simulink model "model"  (R2021a)
settings: Solver=VariableStepAuto  StartTime=0.0  StopTime=50000  RelTol=1e-3
values from neighbouring files (symbols this model uses):
  C_index = 3    [parameters.m]    (also in parameters.mat)
  C_r = 6.6    [parameters.m]    (also in parameters.mat)
  Capacity_noise = 10    [parameters.m]    (also in parameters.mat)
  cell_count = 12    [parameters.m]    (also in parameters.mat)
  Parameter_noise = 80    [parameters.m]    (also in parameters.mat)
  Q_index = 2    [parameters.m]    (also in parameters.mat)
  Rp = Rp_LUT    [parameters.m]    (also in parameters.mat = [0.0013284973182 0.00132849731829 0.00133071540687 0.0013310)
  Rs = Rs_LUT    [parameters.m]    (also in parameters.mat = [0.0044622496006 0.00446224960062 0.00395928973129 0.0036572)
  soc_LUT = [0, 0.01, 0.0909090909090909,0.181818181818182,0.272727272727273,0.363636363636364,0.454545454545455,0.545454545454545,0.636363636363636,0.727272727272727,0.818181818181818,0.909090909090909,1]    [parameters.m]    (also in parameters.mat = [0 0.01 0.0909090909091 0.181818181818 0.272727272727 0.3636)
  tau = tau_LUT    [parameters.m]    (also in parameters.mat = [950.87194683 950.871946837 952.459545918 952.715608142 956.)
  Ts_macro = 60    [parameters.m]    (also in parameters.mat)
  Ts_micro = 0.02    [parameters.m]    (also in parameters.mat)
  z0 = 0.5    [parameters.m]    (also in parameters.mat)
undefined symbols (not defined in the file or in its folder): awgn, CC_level, CV_level, is_CC, is_CV
libraries: nesl_utility x42, fl_lib x30, ee_lib x12, simulink x11, sharedTrackingLibrary x2, simulink_extras x1
(part 1 of 3)
settings Model: SimulationMode=accelerator  Creator=oscar  LastModifiedBy=oscar

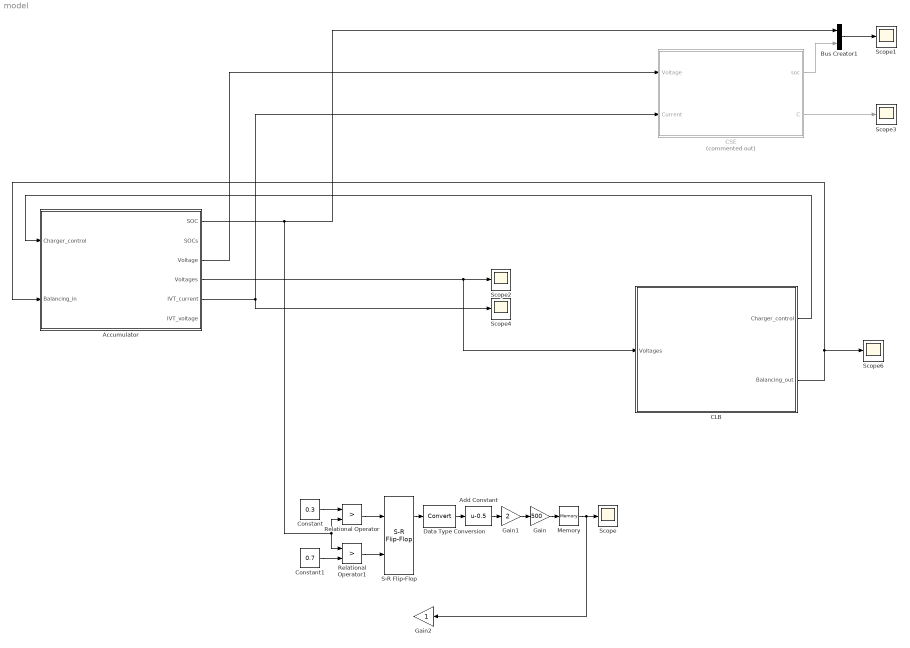
== system model ==
  Accumulator : Subsystem
  Add Constant : Bias  Bias=-0.5
  Bus Creator1 : BusCreator  Inputs=2
  CLB : Subsystem
  CSE : Subsystem  Commented=on
  Constant : Constant  Value=0.3
  Constant1 : Constant  Value=0.7
  Data Type Conversion : DataTypeConversion
  Gain : Gain  Gain=500
  Gain1 : Gain  Gain=2
  Gain2 : Gain
  Memory : Memory
  Relational Operator : RelationalOperator  Operator=>  OutDataTypeStr=boolean  RndMeth=Simplest
  Relational Operator1 : RelationalOperator  Operator=>  OutDataTypeStr=boolean  RndMeth=Simplest
  S-R Flip-Flop : simulink_extras/Flip Flops/S-R Flip-Flop  initial_condition=0
  Scope{,1..4,6} (6 alike) : Scope
  wires:
  Relational Operator/1 -> S-R Flip-Flop/1
  Constant/1 -> Relational Operator/1
  Relational Operator1/1 -> S-R Flip-Flop/2
  Constant1/1 -> Relational Operator1/2
  Accumulator/1(SOC) -> Bus Creator1/1, Relational Operator1/1, Relational Operator/2
  S-R Flip-Flop/1 -> Data Type Conversion/1
  Data Type Conversion/1 -> Add Constant/1
  Gain/1 -> Memory/1
  Memory/1 -> Gain2/1, Scope/1
  Gain1/1 -> Gain/1
  Add Constant/1 -> Gain1/1
  CSE/1(soc) -> Bus Creator1/2
  CSE/2(C) -> Scope3/1
  Accumulator/3(Voltage) -> CSE/1(Voltage)
  Bus Creator1/1 -> Scope1/1
  Accumulator/4(Voltages) -> Scope2/1, CLB/1(Voltages)
  CLB/1(Charger_control) -> Accumulator/1(Charger_control)
  Accumulator/5(IVT_current) -> Scope4/1, CSE/2(Current)
  CLB/2(Balancing_out) -> Scope6/1, Accumulator/2(Balancing_in)

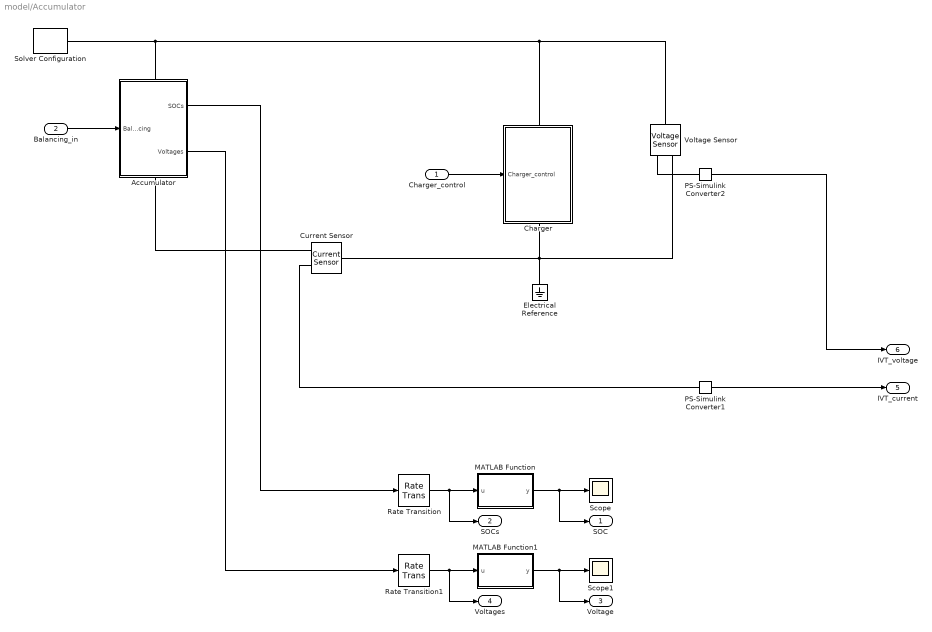
== system model/Accumulator ==
  Charger_control : Inport
  Balancing_in : Inport  Port=2
  Accumulator : Subsystem
      settings: PortSchema="{\"entries\":[{\"content\":{\"sides\":[{\"content\":{\"connectorIds\":[\"In1\"]},\"type\":\"ConnectorPlacement.EquallySpacedRectSide\",\"uuid\":\"7aa37425-1517-42e6-9129-5d9372d372f8\"},{\"content\":{\"connectorIds\":[\"Out1\",\"Out2\"],\"side\":\"RIGHT\"},\"type\":\"ConnectorPlacement.EquallySpacedRectSide\",\"uuid\":\"8265762a-4e80-42de-938c-143734618be7\"},{\"content\":{\"connectorIds\":[\"LConn1\"],\"side\":\"TOP\"},\"type\":\"ConnectorPlacement.EquallySpacedRectSide\",\"uuid\":\"c7d72465-b0c3-4e65-b936-a540327d2954\"},{\"content\":{\"connectorIds\":[\"RConn1\"],\"side\":\"BOTTOM\"},\"type\":\"ConnectorPlacement.EquallySpacedRectSide\",\"uuid\":\"e93312ce-2b0b-47c2-80fe-bdd830a032c3\"}]},\"type\":\"ConnectorPlacement.EquallySpacedConnector\",\"uuid\":\"a59f8eb4-3dec-4028-95ea-1df15449e076\"}],\"packageUris\":[\"http://schema.mathworks.com/mf0/Connector/R2020b\"],\"version\":\"1.0\"}"
  Charger : Subsystem
      settings: PortSchema="{\"entries\":[{\"content\":{\"sides\":[{\"content\":{\"connectorIds\":[\"In1\"]},\"type\":\"ConnectorPlacement.EquallySpacedRectSide\",\"uuid\":\"7aa37425-1517-42e6-9129-5d9372d372f8\"},{\"content\":{\"connectorIds\":[],\"side\":\"RIGHT\"},\"type\":\"ConnectorPlacement.EquallySpacedRectSide\",\"uuid\":\"8265762a-4e80-42de-938c-143734618be7\"},{\"content\":{\"connectorIds\":[\"LConn1\"],\"side\":\"TOP\"},\"type\":\"ConnectorPlacement.EquallySpacedRectSide\",\"uuid\":\"c7d72465-b0c3-4e65-b936-a540327d2954\"},{\"content\":{\"connectorIds\":[\"RConn1\"],\"side\":\"BOTTOM\"},\"type\":\"ConnectorPlacement.EquallySpacedRectSide\",\"uuid\":\"e93312ce-2b0b-47c2-80fe-bdd830a032c3\"}]},\"type\":\"ConnectorPlacement.EquallySpacedConnector\",\"uuid\":\"a59f8eb4-3dec-4028-95ea-1df15449e076\"}],\"packageUris\":[\"http://schema.mathworks.com/mf0/Connector/R2020b\"],\"version\":\"1.0\"}"
  Current Sensor : fl_lib/Electrical/Electrical Sensors/Current Sensor
  Electrical Reference : fl_lib/Electrical/Electrical Elements/Electrical Reference
  MATLAB Function : MATLAB Function  TreatAsAtomicUnit=on
  MATLAB Function1 : MATLAB Function  TreatAsAtomicUnit=on
  PS-Simulink Converter1 : nesl_utility/PS-Simulink Converter  PhysicalDomain=network_engine_domain  SubClassName=ps_output  LeftPortType=input  RightPortType=output  PseudoPeriodic=off  Frequencies=[]  Unit=inherit  AffineConversion=off
      settings: SourceProductBaseCode=PW,SS
  PS-Simulink Converter2 : nesl_utility/PS-Simulink Converter  PhysicalDomain=network_engine_domain  SubClassName=ps_output  LeftPortType=input  RightPortType=output  PseudoPeriodic=off  Frequencies=[]  Unit=inherit  AffineConversion=off
      settings: SourceProductBaseCode=PW,SS
  Rate Transition : RateTransition  OutPortSampleTime=Ts_micro
  Rate Transition1 : RateTransition  OutPortSampleTime=Ts_micro
  Scope : Scope
  Scope1 : Scope
  Solver Configuration : nesl_utility/Solver Configuration  PhysicalDomain=network_engine_domain  SubClassName=solver  LeftPortType=input  RightPortType=generic  Tones=[]  Harmonics=[]  SimulateNoise=off  Profile=off  UseLocalSampling=off  EnableSwitchedLinearOptims=on  FrequencyDomain=off  UseCCode=off  RelTol=0.001  AbsTol=1e-06  MinStep=1e-09  ToWorkspace=off  RevertToSquareIcSolve=off  NumHomotopyIterations=100  PhasorMode=off  PhasorModeNumHarmonics=1  DoDC=off  ResidualTolerance=1e-09  UseLocalSolver=on  LocalSolverChoice=NE_BACKWARD_EULER_ADVANCER  LocalSolverSampleTime=Ts_micro  DoFixedCost=on  MaxNonlinIter=3  MaxModeIter=2  ComputeImpulses=off  ImpulseIterations=2  LinearAlgebra=auto  EquationFormulation=NE_TIME_EF  DelaysMemoryBudget=1024  AutomaticFiltering=on  FilteringTimeConstant=0.001  PartitionStorageMethod=AS_NEEDED  PartitionMemoryBudget=1024  PartitionMethod=ROBUST
      settings: SourceProductBaseCode=PW,SS
  Voltage Sensor : fl_lib/Electrical/Electrical Sensors/Voltage Sensor
  SOC : Outport
  SOCs : Outport  Port=2
  Voltage : Outport  Port=3
  Voltages : Outport  Port=4
  IVT_current : Outport  Port=5
  IVT_voltage : Outport  Port=6
  wires:
  Rate Transition/1 -> MATLAB Function/1(u), SOCs/1
  MATLAB Function/1(y) -> SOC/1, Scope/1
  Rate Transition1/1 -> MATLAB Function1/1(u), Voltages/1
  MATLAB Function1/1(y) -> Scope1/1, Voltage/1
  PS-Simulink Converter1/1 -> IVT_current/1
  PS-Simulink Converter2/1 -> IVT_voltage/1
  Accumulator/2(Voltages) -> Rate Transition1/1
  Accumulator/1(SOCs) -> Rate Transition/1
  Charger_control/1 -> Charger/1(Charger_control)
  Balancing_in/1 -> Accumulator/1(Balancing)
  connections:
  Solver Configuration/RConn1 -- Charger/LConn1 -- Voltage Sensor/LConn1 -- Accumulator/LConn1
  Voltage Sensor/RConn2 -- Current Sensor/LConn1 -- Charger/RConn1 -- Electrical Reference/LConn1
  Accumulator/RConn1 -- Current Sensor/RConn2
  PS-Simulink Converter2/LConn1 -- Voltage Sensor/RConn1
  PS-Simulink Converter1/LConn1 -- Current Sensor/RConn1

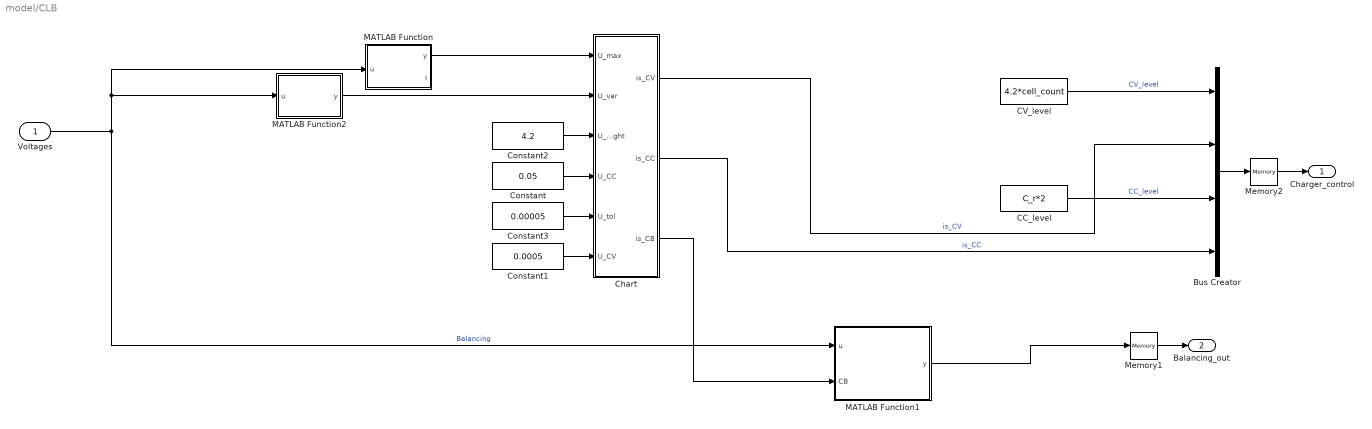
== system model/CLB ==
  Voltages : Inport
  Bus Creator : BusCreator  Inputs=CV_level,is_CV,CC_level,is_CC
  CC_level : Constant  Value=C_r*2
  CV_level : Constant  Value=4.2*cell_count
  Chart : Stateflow chart  TreatAsAtomicUnit=on
  Constant : Constant  Value=0.05
  Constant1 : Constant  Value=0.0005
  Constant2 : Constant  Value=4.2
  Constant3 : Constant  Value=0.00005
  MATLAB Function : MATLAB Function  TreatAsAtomicUnit=on
  MATLAB Function1 : MATLAB Function  TreatAsAtomicUnit=on
  MATLAB Function2 : MATLAB Function  TreatAsAtomicUnit=on
  Memory1 : Memory
  Memory2 : Memory
  Charger_control : Outport
  Balancing_out : Outport  Port=2
  wires:
  Memory2/1 -> Charger_control/1
  CV_level/1 -> Bus Creator/1  "CV_level"
  Bus Creator/1 -> Memory2/1
  CC_level/1 -> Bus Creator/3  "CC_level"
  Memory1/1 -> Balancing_out/1
  MATLAB Function/1(y) -> Chart/1(U_max)
  MATLAB Function2/1(y) -> Chart/2(U_var)
  Constant/1 -> Chart/4(U_CC)
  Constant2/1 -> Chart/3(U_sought)
  Chart/1(is_CV) -> Bus Creator/2  "is_CV"
  Chart/2(is_CC) -> Bus Creator/4  "is_CC"
  Constant1/1 -> Chart/6(U_CV)
  Constant3/1 -> Chart/5(U_tol)
  Voltages/1 -> MATLAB Function1/1(u), MATLAB Function/1(u), MATLAB Function2/1(u)  "Balancing"
  Chart/3(is_CB) -> MATLAB Function1/2(CB)
  MATLAB Function1/1(y) -> Memory1/1

== system model/CSE ==
  Voltage : Inport
  Current : Inport  Port=2
  Subsystem1 : Subsystem
  soc : Outport
  C : Outport  Port=2
  wires:
  Current/1 -> Subsystem1/2(u)  "Measured current"
  Subsystem1/1(soc) -> soc/1
  Voltage/1 -> Subsystem1/1(y)  "Measured terminal voltage"
  Subsystem1/2(C) -> C/1

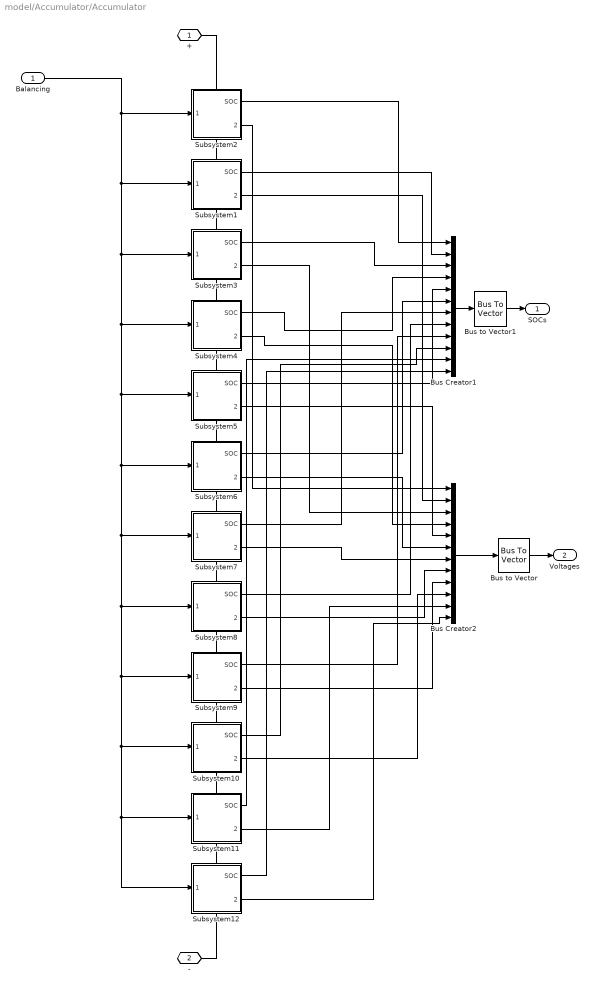
== system model/Accumulator/Accumulator ==
  Balancing : Inport
  Bus Creator1 : BusCreator  Inputs=12
  Bus Creator2 : BusCreator  Inputs=12
  Bus to Vector : BusToVector
  Bus to Vector1 : BusToVector
  Subsystem1 : Subsystem
      settings: PortSchema="{\"entries\":[{\"content\":{\"sides\":[{\"content\":{\"connectorIds\":[\"In1\"]},\"type\":\"ConnectorPlacement.EquallySpacedRectSide\",\"uuid\":\"12454999-d530-49f5-bac0-069dc0ea13eb\"},{\"content\":{\"connectorIds\":[\"Out1\",\"Out2\"],\"side\":\"RIGHT\"},\"type\":\"ConnectorPlacement.EquallySpacedRectSide\",\"uuid\":\"c2464d36-28a6-4c7d-a40d-2467db5248bd\"},{\"content\":{\"connectorIds\":[\"LConn1\"],\"side\":\"TOP\"},\"type\":\"ConnectorPlacement.EquallySpacedRectSide\",\"uuid\":\"cd9dcdbd-9013-49a9-840c-21f78f4a635e\"},{\"content\":{\"connectorIds\":[\"RConn1\"],\"side\":\"BOTTOM\"},\"type\":\"ConnectorPlacement.EquallySpacedRectSide\",\"uuid\":\"e02f0798-3af2-4b56-8f3d-3f1057b9d009\"}]},\"type\":\"ConnectorPlacement.EquallySpacedConnector\",\"uuid\":\"1b50d1f5-ed91-4227-9f31-c0f7430569a7\"}],\"packageUris\":[\"http://schema.mathworks.com/mf0/Connector/R2020b\"],\"version\":\"1.0\"}"
  Subsystem10 : Subsystem
      settings: PortSchema="{\"entries\":[{\"content\":{\"sides\":[{\"content\":{\"connectorIds\":[\"In1\"]},\"type\":\"ConnectorPlacement.EquallySpacedRectSide\",\"uuid\":\"12454999-d530-49f5-bac0-069dc0ea13eb\"},{\"content\":{\"connectorIds\":[\"Out1\",\"Out2\"],\"side\":\"RIGHT\"},\"type\":\"ConnectorPlacement.EquallySpacedRectSide\",\"uuid\":\"c2464d36-28a6-4c7d-a40d-2467db5248bd\"},{\"content\":{\"connectorIds\":[\"LConn1\"],\"side\":\"TOP\"},\"type\":\"ConnectorPlacement.EquallySpacedRectSide\",\"uuid\":\"cd9dcdbd-9013-49a9-840c-21f78f4a635e\"},{\"content\":{\"connectorIds\":[\"RConn1\"],\"side\":\"BOTTOM\"},\"type\":\"ConnectorPlacement.EquallySpacedRectSide\",\"uuid\":\"e02f0798-3af2-4b56-8f3d-3f1057b9d009\"}]},\"type\":\"ConnectorPlacement.EquallySpacedConnector\",\"uuid\":\"1b50d1f5-ed91-4227-9f31-c0f7430569a7\"}],\"packageUris\":[\"http://schema.mathworks.com/mf0/Connector/R2020b\"],\"version\":\"1.0\"}"
  Subsystem11 : Subsystem
      settings: PortSchema="{\"entries\":[{\"content\":{\"sides\":[{\"content\":{\"connectorIds\":[\"In1\"]},\"type\":\"ConnectorPlacement.EquallySpacedRectSide\",\"uuid\":\"12454999-d530-49f5-bac0-069dc0ea13eb\"},{\"content\":{\"connectorIds\":[\"Out1\",\"Out2\"],\"side\":\"RIGHT\"},\"type\":\"ConnectorPlacement.EquallySpacedRectSide\",\"uuid\":\"c2464d36-28a6-4c7d-a40d-2467db5248bd\"},{\"content\":{\"connectorIds\":[\"LConn1\"],\"side\":\"TOP\"},\"type\":\"ConnectorPlacement.EquallySpacedRectSide\",\"uuid\":\"cd9dcdbd-9013-49a9-840c-21f78f4a635e\"},{\"content\":{\"connectorIds\":[\"RConn1\"],\"side\":\"BOTTOM\"},\"type\":\"ConnectorPlacement.EquallySpacedRectSide\",\"uuid\":\"e02f0798-3af2-4b56-8f3d-3f1057b9d009\"}]},\"type\":\"ConnectorPlacement.EquallySpacedConnector\",\"uuid\":\"1b50d1f5-ed91-4227-9f31-c0f7430569a7\"}],\"packageUris\":[\"http://schema.mathworks.com/mf0/Connector/R2020b\"],\"version\":\"1.0\"}"
  Subsystem12 : Subsystem
      settings: PortSchema="{\"entries\":[{\"content\":{\"sides\":[{\"content\":{\"connectorIds\":[\"In1\"]},\"type\":\"ConnectorPlacement.EquallySpacedRectSide\",\"uuid\":\"12454999-d530-49f5-bac0-069dc0ea13eb\"},{\"content\":{\"connectorIds\":[\"Out1\",\"Out2\"],\"side\":\"RIGHT\"},\"type\":\"ConnectorPlacement.EquallySpacedRectSide\",\"uuid\":\"c2464d36-28a6-4c7d-a40d-2467db5248bd\"},{\"content\":{\"connectorIds\":[\"LConn1\"],\"side\":\"TOP\"},\"type\":\"ConnectorPlacement.EquallySpacedRectSide\",\"uuid\":\"cd9dcdbd-9013-49a9-840c-21f78f4a635e\"},{\"content\":{\"connectorIds\":[\"RConn1\"],\"side\":\"BOTTOM\"},\"type\":\"ConnectorPlacement.EquallySpacedRectSide\",\"uuid\":\"e02f0798-3af2-4b56-8f3d-3f1057b9d009\"}]},\"type\":\"ConnectorPlacement.EquallySpacedConnector\",\"uuid\":\"1b50d1f5-ed91-4227-9f31-c0f7430569a7\"}],\"packageUris\":[\"http://schema.mathworks.com/mf0/Connector/R2020b\"],\"version\":\"1.0\"}"
  Subsystem2 : Subsystem
      settings: PortSchema="{\"entries\":[{\"content\":{\"sides\":[{\"content\":{\"connectorIds\":[\"In1\"]},\"type\":\"ConnectorPlacement.EquallySpacedRectSide\",\"uuid\":\"12454999-d530-49f5-bac0-069dc0ea13eb\"},{\"content\":{\"connectorIds\":[\"Out1\",\"Out2\"],\"side\":\"RIGHT\"},\"type\":\"ConnectorPlacement.EquallySpacedRectSide\",\"uuid\":\"c2464d36-28a6-4c7d-a40d-2467db5248bd\"},{\"content\":{\"connectorIds\":[\"LConn1\"],\"side\":\"TOP\"},\"type\":\"ConnectorPlacement.EquallySpacedRectSide\",\"uuid\":\"cd9dcdbd-9013-49a9-840c-21f78f4a635e\"},{\"content\":{\"connectorIds\":[\"RConn1\"],\"side\":\"BOTTOM\"},\"type\":\"ConnectorPlacement.EquallySpacedRectSide\",\"uuid\":\"e02f0798-3af2-4b56-8f3d-3f1057b9d009\"}]},\"type\":\"ConnectorPlacement.EquallySpacedConnector\",\"uuid\":\"1b50d1f5-ed91-4227-9f31-c0f7430569a7\"}],\"packageUris\":[\"http://schema.mathworks.com/mf0/Connector/R2020b\"],\"version\":\"1.0\"}"
  Subsystem3 : Subsystem
      settings: PortSchema="{\"entries\":[{\"content\":{\"sides\":[{\"content\":{\"connectorIds\":[\"In1\"]},\"type\":\"ConnectorPlacement.EquallySpacedRectSide\",\"uuid\":\"12454999-d530-49f5-bac0-069dc0ea13eb\"},{\"content\":{\"connectorIds\":[\"Out1\",\"Out2\"],\"side\":\"RIGHT\"},\"type\":\"ConnectorPlacement.EquallySpacedRectSide\",\"uuid\":\"c2464d36-28a6-4c7d-a40d-2467db5248bd\"},{\"content\":{\"connectorIds\":[\"LConn1\"],\"side\":\"TOP\"},\"type\":\"ConnectorPlacement.EquallySpacedRectSide\",\"uuid\":\"cd9dcdbd-9013-49a9-840c-21f78f4a635e\"},{\"content\":{\"connectorIds\":[\"RConn1\"],\"side\":\"BOTTOM\"},\"type\":\"ConnectorPlacement.EquallySpacedRectSide\",\"uuid\":\"e02f0798-3af2-4b56-8f3d-3f1057b9d009\"}]},\"type\":\"ConnectorPlacement.EquallySpacedConnector\",\"uuid\":\"1b50d1f5-ed91-4227-9f31-c0f7430569a7\"}],\"packageUris\":[\"http://schema.mathworks.com/mf0/Connector/R2020b\"],\"version\":\"1.0\"}"
  Subsystem4 : Subsystem
      settings: PortSchema="{\"entries\":[{\"content\":{\"sides\":[{\"content\":{\"connectorIds\":[\"In1\"]},\"type\":\"ConnectorPlacement.EquallySpacedRectSide\",\"uuid\":\"12454999-d530-49f5-bac0-069dc0ea13eb\"},{\"content\":{\"connectorIds\":[\"Out1\",\"Out2\"],\"side\":\"RIGHT\"},\"type\":\"ConnectorPlacement.EquallySpacedRectSide\",\"uuid\":\"c2464d36-28a6-4c7d-a40d-2467db5248bd\"},{\"content\":{\"connectorIds\":[\"LConn1\"],\"side\":\"TOP\"},\"type\":\"ConnectorPlacement.EquallySpacedRectSide\",\"uuid\":\"cd9dcdbd-9013-49a9-840c-21f78f4a635e\"},{\"content\":{\"connectorIds\":[\"RConn1\"],\"side\":\"BOTTOM\"},\"type\":\"ConnectorPlacement.EquallySpacedRectSide\",\"uuid\":\"e02f0798-3af2-4b56-8f3d-3f1057b9d009\"}]},\"type\":\"ConnectorPlacement.EquallySpacedConnector\",\"uuid\":\"1b50d1f5-ed91-4227-9f31-c0f7430569a7\"}],\"packageUris\":[\"http://schema.mathworks.com/mf0/Connector/R2020b\"],\"version\":\"1.0\"}"
  Subsystem5 : Subsystem
      settings: PortSchema="{\"entries\":[{\"content\":{\"sides\":[{\"content\":{\"connectorIds\":[\"In1\"]},\"type\":\"ConnectorPlacement.EquallySpacedRectSide\",\"uuid\":\"12454999-d530-49f5-bac0-069dc0ea13eb\"},{\"content\":{\"connectorIds\":[\"Out1\",\"Out2\"],\"side\":\"RIGHT\"},\"type\":\"ConnectorPlacement.EquallySpacedRectSide\",\"uuid\":\"c2464d36-28a6-4c7d-a40d-2467db5248bd\"},{\"content\":{\"connectorIds\":[\"LConn1\"],\"side\":\"TOP\"},\"type\":\"ConnectorPlacement.EquallySpacedRectSide\",\"uuid\":\"cd9dcdbd-9013-49a9-840c-21f78f4a635e\"},{\"content\":{\"connectorIds\":[\"RConn1\"],\"side\":\"BOTTOM\"},\"type\":\"ConnectorPlacement.EquallySpacedRectSide\",\"uuid\":\"e02f0798-3af2-4b56-8f3d-3f1057b9d009\"}]},\"type\":\"ConnectorPlacement.EquallySpacedConnector\",\"uuid\":\"1b50d1f5-ed91-4227-9f31-c0f7430569a7\"}],\"packageUris\":[\"http://schema.mathworks.com/mf0/Connector/R2020b\"],\"version\":\"1.0\"}"
  Subsystem6 : Subsystem
      settings: PortSchema="{\"entries\":[{\"content\":{\"sides\":[{\"content\":{\"connectorIds\":[\"In1\"]},\"type\":\"ConnectorPlacement.EquallySpacedRectSide\",\"uuid\":\"12454999-d530-49f5-bac0-069dc0ea13eb\"},{\"content\":{\"connectorIds\":[\"Out1\",\"Out2\"],\"side\":\"RIGHT\"},\"type\":\"ConnectorPlacement.EquallySpacedRectSide\",\"uuid\":\"c2464d36-28a6-4c7d-a40d-2467db5248bd\"},{\"content\":{\"connectorIds\":[\"LConn1\"],\"side\":\"TOP\"},\"type\":\"ConnectorPlacement.EquallySpacedRectSide\",\"uuid\":\"cd9dcdbd-9013-49a9-840c-21f78f4a635e\"},{\"content\":{\"connectorIds\":[\"RConn1\"],\"side\":\"BOTTOM\"},\"type\":\"ConnectorPlacement.EquallySpacedRectSide\",\"uuid\":\"e02f0798-3af2-4b56-8f3d-3f1057b9d009\"}]},\"type\":\"ConnectorPlacement.EquallySpacedConnector\",\"uuid\":\"1b50d1f5-ed91-4227-9f31-c0f7430569a7\"}],\"packageUris\":[\"http://schema.mathworks.com/mf0/Connector/R2020b\"],\"version\":\"1.0\"}"
  Subsystem7 : Subsystem
      settings: PortSchema="{\"entries\":[{\"content\":{\"sides\":[{\"content\":{\"connectorIds\":[\"In1\"]},\"type\":\"ConnectorPlacement.EquallySpacedRectSide\",\"uuid\":\"12454999-d530-49f5-bac0-069dc0ea13eb\"},{\"content\":{\"connectorIds\":[\"Out1\",\"Out2\"],\"side\":\"RIGHT\"},\"type\":\"ConnectorPlacement.EquallySpacedRectSide\",\"uuid\":\"c2464d36-28a6-4c7d-a40d-2467db5248bd\"},{\"content\":{\"connectorIds\":[\"LConn1\"],\"side\":\"TOP\"},\"type\":\"ConnectorPlacement.EquallySpacedRectSide\",\"uuid\":\"cd9dcdbd-9013-49a9-840c-21f78f4a635e\"},{\"content\":{\"connectorIds\":[\"RConn1\"],\"side\":\"BOTTOM\"},\"type\":\"ConnectorPlacement.EquallySpacedRectSide\",\"uuid\":\"e02f0798-3af2-4b56-8f3d-3f1057b9d009\"}]},\"type\":\"ConnectorPlacement.EquallySpacedConnector\",\"uuid\":\"1b50d1f5-ed91-4227-9f31-c0f7430569a7\"}],\"packageUris\":[\"http://schema.mathworks.com/mf0/Connector/R2020b\"],\"version\":\"1.0\"}"
  Subsystem8 : Subsystem
      settings: PortSchema="{\"entries\":[{\"content\":{\"sides\":[{\"content\":{\"connectorIds\":[\"In1\"]},\"type\":\"ConnectorPlacement.EquallySpacedRectSide\",\"uuid\":\"12454999-d530-49f5-bac0-069dc0ea13eb\"},{\"content\":{\"connectorIds\":[\"Out1\",\"Out2\"],\"side\":\"RIGHT\"},\"type\":\"ConnectorPlacement.EquallySpacedRectSide\",\"uuid\":\"c2464d36-28a6-4c7d-a40d-2467db5248bd\"},{\"content\":{\"connectorIds\":[\"LConn1\"],\"side\":\"TOP\"},\"type\":\"ConnectorPlacement.EquallySpacedRectSide\",\"uuid\":\"cd9dcdbd-9013-49a9-840c-21f78f4a635e\"},{\"content\":{\"connectorIds\":[\"RConn1\"],\"side\":\"BOTTOM\"},\"type\":\"ConnectorPlacement.EquallySpacedRectSide\",\"uuid\":\"e02f0798-3af2-4b56-8f3d-3f1057b9d009\"}]},\"type\":\"ConnectorPlacement.EquallySpacedConnector\",\"uuid\":\"1b50d1f5-ed91-4227-9f31-c0f7430569a7\"}],\"packageUris\":[\"http://schema.mathworks.com/mf0/Connector/R2020b\"],\"version\":\"1.0\"}"
  Subsystem9 : Subsystem
      settings: PortSchema="{\"entries\":[{\"content\":{\"sides\":[{\"content\":{\"connectorIds\":[\"In1\"]},\"type\":\"ConnectorPlacement.EquallySpacedRectSide\",\"uuid\":\"12454999-d530-49f5-bac0-069dc0ea13eb\"},{\"content\":{\"connectorIds\":[\"Out1\",\"Out2\"],\"side\":\"RIGHT\"},\"type\":\"ConnectorPlacement.EquallySpacedRectSide\",\"uuid\":\"c2464d36-28a6-4c7d-a40d-2467db5248bd\"},{\"content\":{\"connectorIds\":[\"LConn1\"],\"side\":\"TOP\"},\"type\":\"ConnectorPlacement.EquallySpacedRectSide\",\"uuid\":\"cd9dcdbd-9013-49a9-840c-21f78f4a635e\"},{\"content\":{\"connectorIds\":[\"RConn1\"],\"side\":\"BOTTOM\"},\"type\":\"ConnectorPlacement.EquallySpacedRectSide\",\"uuid\":\"e02f0798-3af2-4b56-8f3d-3f1057b9d009\"}]},\"type\":\"ConnectorPlacement.EquallySpacedConnector\",\"uuid\":\"1b50d1f5-ed91-4227-9f31-c0f7430569a7\"}],\"packageUris\":[\"http://schema.mathworks.com/mf0/Connector/R2020b\"],\"version\":\"1.0\"}"
  + : PMIOPort  Side=Left
  - : PMIOPort  Port=2  Side=Right
  SOCs : Outport
  Voltages : Outport  Port=2
  wires:
  Balancing/1 -> Subsystem12/1(Balance), Subsystem11/1(Balance), Subsystem10/1(Balance), Subsystem9/1(Balance), Subsystem8/1(Balance), Subsystem7/1(Balance), Subsystem6/1(Balance), Subsystem5/1(Balance), Subsystem4/1(Balance), Subsystem3/1(Balance), Subsystem1/1(Balance), Subsystem2/1(Balance)
  Bus Creator2/1 -> Bus to Vector/1
  Bus to Vector/1 -> Voltages/1
  Bus to Vector1/1 -> SOCs/1
  Bus Creator1/1 -> Bus to Vector1/1
  Subsystem2/1(SOC) -> Bus Creator1/1
  Subsystem1/1(SOC) -> Bus Creator1/2
  Subsystem3/1(SOC) -> Bus Creator1/3
  Subsystem4/1(SOC) -> Bus Creator1/4
  Subsystem5/1(SOC) -> Bus Creator1/5
  Subsystem6/1(SOC) -> Bus Creator1/6
  Subsystem7/1(SOC) -> Bus Creator1/7
  Subsystem8/1(SOC) -> Bus Creator1/8
  Subsystem9/1(SOC) -> Bus Creator1/9
  Subsystem10/1(SOC) -> Bus Creator1/10
  Subsystem11/1(SOC) -> Bus Creator1/11
  Subsystem12/1(SOC) -> Bus Creator1/12
  Subsystem2/2(Voltage) -> Bus Creator2/1
  Subsystem1/2(Voltage) -> Bus Creator2/2
  Subsystem3/2(Voltage) -> Bus Creator2/3
  Subsystem4/2(Voltage) -> Bus Creator2/4
  Subsystem5/2(Voltage) -> Bus Creator2/5
  Subsystem6/2(Voltage) -> Bus Creator2/6
  Subsystem7/2(Voltage) -> Bus Creator2/7
  Subsystem8/2(Voltage) -> Bus Creator2/8
  Subsystem9/2(Voltage) -> Bus Creator2/9
  Subsystem10/2(Voltage) -> Bus Creator2/10
  Subsystem11/2(Voltage) -> Bus Creator2/11
  Subsystem12/2(Voltage) -> Bus Creator2/12
  connections:
  Subsystem2/LConn1 -- +/RConn1
  Subsystem12/RConn1 -- -/RConn1
  Subsystem1/LConn1 -- Subsystem2/RConn1
  Subsystem4/LConn1 -- Subsystem3/RConn1
  Subsystem5/LConn1 -- Subsystem4/RConn1
  Subsystem6/LConn1 -- Subsystem5/RConn1
  Subsystem7/LConn1 -- Subsystem6/RConn1
  Subsystem7/RConn1 -- Subsystem8/LConn1
  Subsystem11/LConn1 -- Subsystem10/RConn1
  Subsystem10/LConn1 -- Subsystem9/RConn1
  Subsystem11/RConn1 -- Subsystem12/LConn1
  Subsystem8/RConn1 -- Subsystem9/LConn1
  Subsystem1/RConn1 -- Subsystem3/LConn1

== system model/Accumulator/Charger ==
  Charger_control : Inport
  Bus Selector : BusSelector  OutputSignals=CV_level,is_CV,CC_level,is_CC
  Controlled Current Source : fl_lib/Electrical/Electrical Sources/Controlled Current Source
  Controlled Voltage Source : fl_lib/Electrical/Electrical Sources/Controlled Voltage Source
  Product : Product
  Simulink-PS Converter1 : nesl_utility/Simulink-PS Converter  PhysicalDomain=network_engine_domain  SubClassName=ps_input  LeftPortType=input  RightPortType=output  PseudoPeriodic=off  Frequencies=[]  NoiseDistribution=none  NoiseParameters=[]  Unit=1  AffineConversion=off  FilteringAndDerivatives=provide  SimscapeFilterOrder=1  InputFilterTimeConstant=0.001  UdotUserProvided=0
      settings: SourceProductBaseCode=PW,SS
  Simulink-PS Converter2 : nesl_utility/Simulink-PS Converter  PhysicalDomain=network_engine_domain  SubClassName=ps_input  LeftPortType=input  RightPortType=output  PseudoPeriodic=off  Frequencies=[]  NoiseDistribution=none  NoiseParameters=[]  Unit=1  AffineConversion=off  FilteringAndDerivatives=provide  SimscapeFilterOrder=1  InputFilterTimeConstant=0.001  UdotUserProvided=0
      settings: SourceProductBaseCode=PW,SS
  Simulink-PS Converter4 : nesl_utility/Simulink-PS Converter  PhysicalDomain=network_engine_domain  SubClassName=ps_input  LeftPortType=input  RightPortType=output  PseudoPeriodic=off  Frequencies=[]  NoiseDistribution=none  NoiseParameters=[]  Unit=1  AffineConversion=off  FilteringAndDerivatives=provide  SimscapeFilterOrder=1  InputFilterTimeConstant=0.001  UdotUserProvided=0
      settings: SourceProductBaseCode=PW,SS
  Switch : fl_lib/Electrical/Electrical Elements/Switch  R_closed=0.01 Ohm  G_open=1e-33 1/Ohm  Threshold=0.5  i_specify=off  i_priority=None  i=0 A  i_nominal_specify=off  i_nominal_unit=A  i_nominal_value=1  v_specify=off  v_priority=None  v=0 V  v_nominal_specify=off  v_nominal_unit=V  v_nominal_value=1
  + : PMIOPort  Side=Left
  - : PMIOPort  Port=2  Side=Right
  wires:
  Charger_control/1 -> Bus Selector/1
  Bus Selector/1 -> Simulink-PS Converter2/1  "<CV_level>"
  Bus Selector/2 -> Simulink-PS Converter1/1  "<is_CV>"
  Bus Selector/4 -> Product/2  "<is_CC>"
  Bus Selector/3 -> Product/1  "<CC_level>"
  Product/1 -> Simulink-PS Converter4/1
  connections:
  Switch/RConn1 -- Simulink-PS Converter1/RConn1
  Controlled Voltage Source/LConn1 -- +/RConn1 -- Controlled Current Source/LConn1
  Controlled Voltage Source/RConn1 -- Simulink-PS Converter2/RConn1
  Switch/LConn1 -- Controlled Voltage Source/RConn2
  Switch/RConn2 -- Controlled Current Source/RConn2 -- -/RConn1
  Simulink-PS Converter4/RConn1 -- Controlled Current Source/RConn1

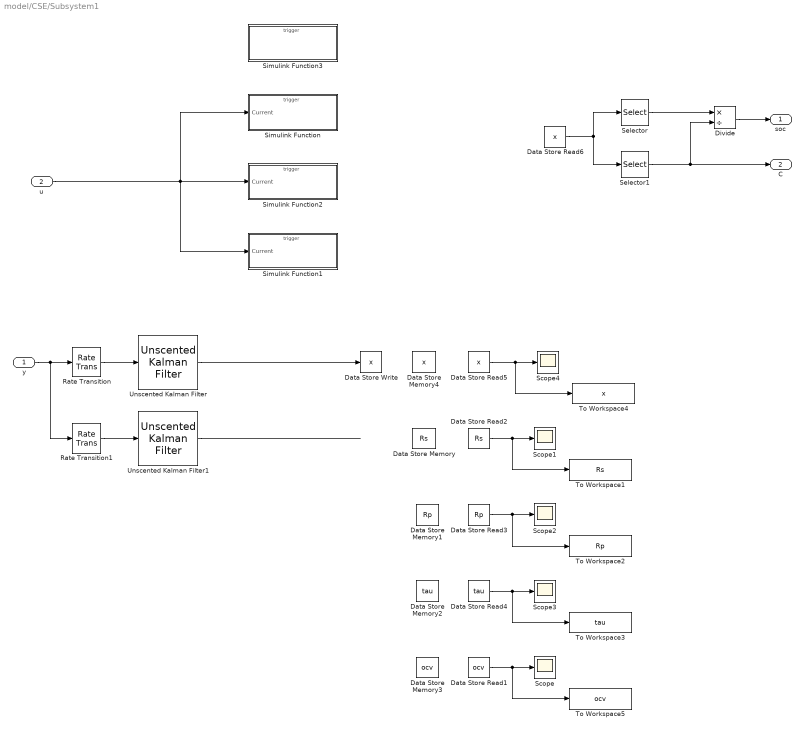
== system model/CSE/Subsystem1 ==
  y : Inport
  u : Inport  Port=2
  Data Store Memory : DataStoreMemory  DataStoreName=Rs  ReadBeforeWriteMsg=warning  WriteAfterWriteMsg=warning  WriteAfterReadMsg=warning  InitialValue=Rs_LUT  ShowAdditionalParam=off
  Data Store Memory1 : DataStoreMemory  DataStoreName=Rp  ReadBeforeWriteMsg=warning  WriteAfterWriteMsg=warning  WriteAfterReadMsg=warning  InitialValue=Rp_LUT  ShowAdditionalParam=off
  Data Store Memory2 : DataStoreMemory  DataStoreName=tau  ReadBeforeWriteMsg=warning  WriteAfterWriteMsg=warning  WriteAfterReadMsg=warning  InitialValue=tau_LUT  ShowAdditionalParam=off
  Data Store Memory3 : DataStoreMemory  DataStoreName=ocv  ReadBeforeWriteMsg=warning  WriteAfterWriteMsg=warning  WriteAfterReadMsg=warning  InitialValue=ocv_LUT  ShowAdditionalParam=off
  Data Store Memory4 : DataStoreMemory  DataStoreName=x  ReadBeforeWriteMsg=warning  WriteAfterWriteMsg=warning  WriteAfterReadMsg=warning  InitialValue=x0  ShowAdditionalParam=off
  Data Store Read1 : DataStoreRead  DataStoreName=ocv  IndexOptions=Index vector (dialog)  Indices=1  OutputSizes=1
  Data Store Read2 : DataStoreRead  DataStoreName=Rs  IndexOptions=Index vector (dialog)  Indices=1  OutputSizes=1
  Data Store Read3 : DataStoreRead  DataStoreName=Rp  IndexOptions=Index vector (dialog)  Indices=1  OutputSizes=1
  Data Store Read4 : DataStoreRead  DataStoreName=tau  IndexOptions=Index vector (dialog)  Indices=1  OutputSizes=1
  Data Store Read5 : DataStoreRead  DataStoreName=x  IndexOptions=Index vector (dialog)  Indices=1  OutputSizes=1
  Data Store Read6 : DataStoreRead  DataStoreName=x  IndexOptions=Index vector (dialog)  Indices=1  OutputSizes=1
  Data Store Write : DataStoreWrite  DataStoreName=x  IndexOptions=Index vector (dialog)  Indices=1  OutputSizes=1
  Divide : Product  Inputs=*/
  Rate Transition : RateTransition  OutPortSampleTime=Ts_micro
  Rate Transition1 : RateTransition  OutPortSampleTime=Ts_macro
  Scope{,1..4} (5 alike) : Scope
  Selector : Selector  InputPortWidth=l_x  IndexOptions=Index vector (dialog)  Indices=[Q_index]  OutputSizes=1
  Selector1 : Selector  InputPortWidth=l_x  IndexOptions=Index vector (dialog)  Indices=[C_index]  OutputSizes=1
  Simulink Function : Subsystem  TreatAsAtomicUnit=on
  Simulink Function1 : Subsystem  TreatAsAtomicUnit=on
  Simulink Function2 : Subsystem  TreatAsAtomicUnit=on
  Simulink Function3 : Subsystem  TreatAsAtomicUnit=on
  To Workspace1 : ToWorkspace  VariableName=Rs  SampleTime=-1
      settings: MaxDataPoints=1
  To Workspace2 : ToWorkspace  VariableName=Rp  SampleTime=-1
      settings: MaxDataPoints=1
  To Workspace3 : ToWorkspace  VariableName=tau  SampleTime=-1
      settings: MaxDataPoints=1
  To Workspace4 : ToWorkspace  VariableName=x  SampleTime=-1
      settings: MaxDataPoints=1
  To Workspace5 : ToWorkspace  VariableName=ocv  SampleTime=-1
      settings: MaxDataPoints=1
  Unscented Kalman Filter : sharedTrackingLibrary/Unscented Kalman Filter  StateTransitionFcn=S_x  HasAdditiveProcessNoise=Additive  ProcessNoise=Px0  HasTimeVaryingProcessNoise=off  HasStateTransitionFcnExtraArgument=0  InitialState=x0  InitialStateCovariance=Qx0  Alpha=0.2  Beta=2  Kappa=0  MeasurementFcn1=M_x  HasMeasurementEnablePort1=off  HasAdditiveMeasurementNoise1=Additive  MeasurementNoise1=Rx0  HasTimeVaryingMeasurementNoise1=off  HasMeasurementFcnExtraArgument1=0  MeasurementFcn2=myMeasurementFcn  HasMeasurementEnablePort2=off  HasAdditiveMeasurementNoise2=Additive  MeasurementNoise2=1  HasTimeVaryingMeasurementNoise2=off  HasMeasurementFcnExtraArgument2=0  MeasurementFcn3=myMeasurementFcn  HasMeasurementEnablePort3=off  HasAdditiveMeasurementNoise3=Additive  MeasurementNoise3=1  HasTimeVaryingMeasurementNoise3=off  HasMeasurementFcnExtraArgument3=0  MeasurementFcn4=myMeasurementFcn  HasMeasurementEnablePort4=off  HasAdditiveMeasurementNoise4=Additive  MeasurementNoise4=1  HasTimeVaryingMeasurementNoise4=off  HasMeasurementFcnExtraArgument4=0  MeasurementFcn5=myMeasurementFcn  HasMeasurementEnablePort5=off  HasAdditiveMeasurementNoise5=Additive  MeasurementNoise5=1  HasTimeVaryingMeasurementNoise5=off  HasMeasurementFcnExtraArgument5=0  EnableMultirate=off  StateTransitionFcnSampleTime=1  MeasurementFcn1SampleTime=1  MeasurementFcn2SampleTime=1  MeasurementFcn3SampleTime=1  MeasurementFcn4SampleTime=1  MeasurementFcn5SampleTime=1  UseCurrentEstimator=on  OutputStateCovariance=off  DataType=double  SampleTime=Ts_micro  NumberOfMeasurements=1
      settings: SourceProductBaseCode=CT,DR,TF,ID,LP,NV,AR,RO,RR,UV,VE
  Unscented Kalman Filter1 : sharedTrackingLibrary/Unscented Kalman Filter  StateTransitionFcn=S_p  HasAdditiveProcessNoise=Additive  ProcessNoise=1e-7*diag(Rs)  HasTimeVaryingProcessNoise=off  HasStateTransitionFcnExtraArgument=0  InitialState=Rs  InitialStateCovariance=1e-7*diag(Rs)  Alpha=0.2  Beta=2  Kappa=0  MeasurementFcn1=M_Rs  HasMeasurementEnablePort1=off  HasAdditiveMeasurementNoise1=Additive  MeasurementNoise1=1e-4  HasTimeVaryingMeasurementNoise1=off  HasMeasurementFcnExtraArgument1=0  MeasurementFcn2=myMeasurementFcn  HasMeasurementEnablePort2=off  HasAdditiveMeasurementNoise2=Additive  MeasurementNoise2=1  HasTimeVaryingMeasurementNoise2=off  HasMeasurementFcnExtraArgument2=0  MeasurementFcn3=myMeasurementFcn  HasMeasurementEnablePort3=off  HasAdditiveMeasurementNoise3=Additive  MeasurementNoise3=1  HasTimeVaryingMeasurementNoise3=off  HasMeasurementFcnExtraArgument3=0  MeasurementFcn4=myMeasurementFcn  HasMeasurementEnablePort4=off  HasAdditiveMeasurementNoise4=Additive  MeasurementNoise4=1  HasTimeVaryingMeasurementNoise4=off  HasMeasurementFcnExtraArgument4=0  MeasurementFcn5=myMeasurementFcn  HasMeasurementEnablePort5=off  HasAdditiveMeasurementNoise5=Additive  MeasurementNoise5=1  HasTimeVaryingMeasurementNoise5=off  HasMeasurementFcnExtraArgument5=0  EnableMultirate=off  StateTransitionFcnSampleTime=1  MeasurementFcn1SampleTime=1  MeasurementFcn2SampleTime=1  MeasurementFcn3SampleTime=1  MeasurementFcn4SampleTime=1  MeasurementFcn5SampleTime=1  UseCurrentEstimator=on  OutputStateCovariance=off  DataType=double  SampleTime=Ts_macro  NumberOfMeasurements=1
      settings: SourceProductBaseCode=CT,DR,TF,ID,LP,NV,AR,RO,RR,UV,VE
  soc : Outport
  C : Outport  Port=2
  wires:
  Unscented Kalman Filter/1 -> Data Store Write/1
  Rate Transition/1 -> Unscented Kalman Filter/1
  Data Store Read2/1 -> To Workspace1/1, Scope1/1
  Data Store Read3/1 -> To Workspace2/1, Scope2/1
  Data Store Read4/1 -> To Workspace3/1, Scope3/1
  Selector1/1 -> C/1, Divide/2
  Selector/1 -> Divide/1
  Divide/1 -> soc/1
  Data Store Read6/1 -> Selector1/1, Selector/1
  Data Store Read5/1 -> To Workspace4/1, Scope4/1
  Data Store Read1/1 -> Scope/1, To Workspace5/1
  u/1 -> Simulink Function2/1(Current), Simulink Function1/1(Current), Simulink Function/1(Current)
  Rate Transition1/1 -> Unscented Kalman Filter1/1
  Unscented Kalman Filter1/1 -> ?
  y/1 -> Rate Transition1/1, Rate Transition/1

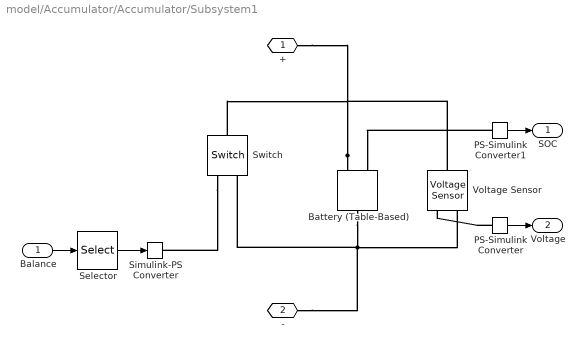
== system model/Accumulator/Accumulator/Subsystem1 ==
  Balance : Inport
  Battery (Table-Based) : ee_lib/Sources/Battery (Table-Based)  SOC_vec=soc_LUT  T_dependence=ee.enum.temperature_dependence.no  prm_dir=ee.enum.battery.prm_dir.noCurrentDirectionality  T_vec=[273.15, 298.15, 323.15] K  V0_mat=[3.2, 3.1, 3.14; 3.25, 3.27, 3.3; 3.28, 3.31, 3.34; 3.33, 3.5, 3.59] V  V0_vec=ocv_LUT V  R0_mat=[.03, .015, .002; .04, .017, .008; .039, .012, .006; .027, .013, .021] Ohm  R0_vec=awgn(Rs, Parameter_noise) Ohm  R0_dis_mat=[.03, .015, .002; .04, .017, .008; .039, .012, .006; .027, .013, .021] Ohm  R0_dis_vec=[.015, .017, .012, .013] Ohm  R0_ch_mat=[.03, .015, .002; .04, .017, .008; .039, .012, .006; .027, .013, .021] Ohm  R0_ch_vec=[.015, .017, .012, .013] Ohm  AH_vec=[2.9, 4.1, 4.2] hr*A  AH=awgn(C_r, Capacity_noise) hr*A  prm_leak=ee.enum.battery.prm_leak.disabled  Rleak_vec=[8000, 7000, 6000] Ohm  Rleak=7e3 Ohm  extrapolation_option=ee.enum.extrapolation.linear  prm_dyn=ee.enum.battery.prm_dyn.rc1  R1_mat=[.089, .076, .01; .042, .022, .099; .019, .007, .002; .051, .043, .029] Ohm  R1_vec=awgn(Rp, Parameter_noise) Ohm  tau1_mat=[44, 148, 235; 93, 110, 1000; 19, 27, 133; .5, 22, 3] s  tau1_vec=awgn(tau, Parameter_noise) s  R2_mat=[.014, .382, .407; .028, .006, .007; .014, .007, .006; .333, .956, .912] Ohm  R2_vec=[.382, .006, .007, .956] Ohm  tau2_mat=[1, 44, 5644; 11, 24, 506; 2, 14, 330; 3310, 13419, 30216] s  tau2_vec=[44, 24, 14, 13419] s  R3_mat=[.014, .382, .407; .028, .006, .007; .014, .007, .006; .333, .956, .912] Ohm  R3_vec=[.382, .006, .007, .956] Ohm  tau3_mat=[1, 44, 5644; 11, 24, 506; 2, 14, 330; 3310, 13419, 30216] s  tau3_vec=[44, 24, 14, 13419] s  R4_mat=[.014, .382, .407; .028, .006, .007; .014, .007, .006; .333, .956, .912] Ohm  R4_vec=[.382, .006, .007, .956] Ohm  tau4_mat=[1, 44, 5644; 11, 24, 506; 2, 14, 330; 3310, 13419, 30216] s  tau4_vec=[44, 24, 14, 13419] s  R5_mat=[.014, .382, .407; .028, .006, .007; .014, .007, .006; .333, .956, .912] Ohm  R5_vec=[.382, .006, .007, .956] Ohm  tau5_mat=[1, 44, 5644; 11, 24, 506; 2, 14, 330; 3310, 13419, 30216] s  tau5_vec=[44, 24, 14, 13419] s  prm_fade=ee.enum.battery.prm_fade.equations  N0=10  dV0=0  dR0=0  dAH=Capacity_deterioration  dRleak=0  dR1=0  dR2=0  dR3=0  dR4=0  dR5=0  N0vec=[100, 200, 300]  Tfadevec=[298.15, 323.15] K  dV0vec=[0, 0, 0]  dR0vec=[0, 0, 0]  dAHvec=[0, 0, 0]  dRleakvec=[0, 0, 0]  dR1vec=[0, 0, 0]  dR2vec=[0, 0, 0]  dR3vec=[0, 0, 0]  dR4vec=[0, 0, 0]  dR5vec=[0, 0, 0]  dV0mat=[0, 0; 0, 0; 0, 0]  dR0mat=[0, 0; 0, 0; 0, 0]  dAHmat=[0, 0; 0, 0; 0, 0]  dRleakmat=[0, 0; 0, 0; 0, 0]  dR1mat=[0, 0; 0, 0; 0, 0]  dR2mat=[0, 0; 0, 0; 0, 0]  dR3mat=[0, 0; 0, 0; 0, 0]  dR4mat=[0, 0; 0, 0; 0, 0]  dR5mat=[0, 0; 0, 0; 0, 0]  prm_age=ee.enum.battery.prm_age.disabled  prm_age_OCV=ee.enum.battery.prm_age_OCV.OCV  OCV_age=0.9  SOC_age=0.6  storage_dt_age_vec=[0] d  storage_T_age_vec=[273] K  OCV_scaling_age=2.2134e6  OCV_offset_age=1.632e6  temp_exp_age=0.515833569 V  t_exp_age=0.75  T_age_vec=[273.15, 298.15, 323.15] K  dt_age_vec=[90, 180, 270, 360] d  dR0_age_vec=[0, 0, 0]  t_meas_dR0_age=100 d  dR0_age_mat=[0, 0, 0; 0, 0, 0; 0, 0, 0; 0, 0, 0]  temperature=298.15 K  i_specify=off  i_priority=None  i=0 A  i_nominal_specify=off  i_nominal_unit=A  i_nominal_value=1  v_specify=off  v_priority=None  v=0 V  v_nominal_specify=off  v_nominal_unit=V  v_nominal_value=1  stateOfCharge_specify=on  stateOfCharge_priority=High  stateOfCharge=z0*1.3  stateOfCharge_nominal_specify=off  stateOfCharge_nominal_unit=1  stateOfCharge_nominal_value=1  num_cycles_specify=off  num_cycles_priority=High  num_cycles=0  num_cycles_nominal_specify=off  num_cycles_nominal_unit=1  num_cycles_nominal_value=1  thermal_mass=30000 J/K  temperature_specify=off  temperature_priority=High  temperature_nominal_specify=off  temperature_nominal_unit=K  temperature_nominal_value=1
      settings: SourceProductBaseCode=PS  InternalSimscapePortConfiguration="{\"Bottom\":[],\"Left\":[{\"id\":\"p\",\"label\":\"+\",\"type\":\"foundation.electrical.electrical\"},{\"id\":\"soc\",\"label\":\"SOC\",\"type\":\"output\"}],\"Right\":[{\"id\":\"n\",\"label\":\"-\",\"type\":\"foundation.electrical.electrical\"}],\"Top\":[]}"
  PS-Simulink Converter : nesl_utility/PS-Simulink Converter  PhysicalDomain=network_engine_domain  SubClassName=ps_output  LeftPortType=input  RightPortType=output  PseudoPeriodic=off  Frequencies=[]  Unit=inherit  AffineConversion=off
      settings: SourceProductBaseCode=PW,SS
  PS-Simulink Converter1 : nesl_utility/PS-Simulink Converter  PhysicalDomain=network_engine_domain  SubClassName=ps_output  LeftPortType=input  RightPortType=output  PseudoPeriodic=off  Frequencies=[]  Unit=inherit  AffineConversion=off
      settings: SourceProductBaseCode=PW,SS
  Selector : Selector  InputPortWidth=cell_count  IndexOptions=Index vector (dialog)  Indices=2  OutputSizes=1
  Simulink-PS Converter : nesl_utility/Simulink-PS Converter  PhysicalDomain=network_engine_domain  SubClassName=ps_input  LeftPortType=input  RightPortType=output  PseudoPeriodic=off  Frequencies=[]  NoiseDistribution=none  NoiseParameters=[]  Unit=1  AffineConversion=off  FilteringAndDerivatives=provide  SimscapeFilterOrder=1  InputFilterTimeConstant=0.001  UdotUserProvided=0
      settings: SourceProductBaseCode=PW,SS
  Switch : fl_lib/Electrical/Electrical Elements/Switch  R_closed=33 Ohm  G_open=1e-8 1/Ohm  Threshold=0.5  i_specify=off  i_priority=None  i=0 A  i_nominal_specify=off  i_nominal_unit=A  i_nominal_value=1  v_specify=off  v_priority=None  v=0 V  v_nominal_specify=off  v_nominal_unit=V  v_nominal_value=1
  Voltage Sensor : fl_lib/Electrical/Electrical Sensors/Voltage Sensor
  + : PMIOPort  Side=Left
  - : PMIOPort  Port=2  Side=Right
  SOC : Outport
  Voltage : Outport  Port=2
  wires:
  PS-Simulink Converter1/1 -> SOC/1
  PS-Simulink Converter/1 -> Voltage/1
  Balance/1 -> Selector/1
  Selector/1 -> Simulink-PS Converter/1
  connections:
  Battery (Table-Based)/LConn1 -- +/RConn1 -- Voltage Sensor/LConn1 -- Switch/LConn1
  PS-Simulink Converter/LConn1 -- Voltage Sensor/RConn1
  PS-Simulink Converter1/LConn1 -- Battery (Table-Based)/LConn2
  Battery (Table-Based)/RConn1 -- Switch/RConn2 -- -/RConn1 -- Voltage Sensor/RConn2
  Switch/RConn1 -- Simulink-PS Converter/RConn1

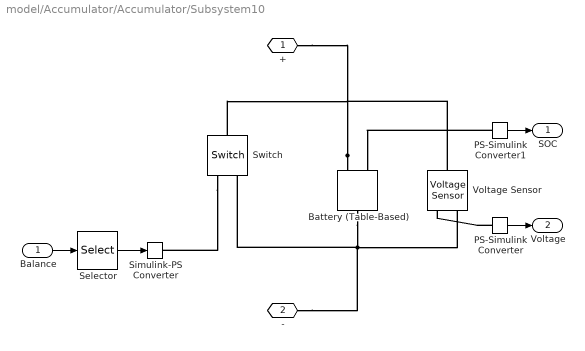
== system model/Accumulator/Accumulator/Subsystem10 ==
  Balance : Inport
  Battery (Table-Based) : ee_lib/Sources/Battery (Table-Based)  SOC_vec=soc_LUT  T_dependence=ee.enum.temperature_dependence.no  prm_dir=ee.enum.battery.prm_dir.noCurrentDirectionality  T_vec=[273.15, 298.15, 323.15] K  V0_mat=[3.2, 3.1, 3.14; 3.25, 3.27, 3.3; 3.28, 3.31, 3.34; 3.33, 3.5, 3.59] V  V0_vec=ocv_LUT V  R0_mat=[.03, .015, .002; .04, .017, .008; .039, .012, .006; .027, .013, .021] Ohm  R0_vec=awgn(Rs, Parameter_noise) Ohm  R0_dis_mat=[.03, .015, .002; .04, .017, .008; .039, .012, .006; .027, .013, .021] Ohm  R0_dis_vec=[.015, .017, .012, .013] Ohm  R0_ch_mat=[.03, .015, .002; .04, .017, .008; .039, .012, .006; .027, .013, .021] Ohm  R0_ch_vec=[.015, .017, .012, .013] Ohm  AH_vec=[2.9, 4.1, 4.2] hr*A  AH=awgn(C_r, Capacity_noise) hr*A  prm_leak=ee.enum.battery.prm_leak.disabled  Rleak_vec=[8000, 7000, 6000] Ohm  Rleak=7e3 Ohm  extrapolation_option=ee.enum.extrapolation.linear  prm_dyn=ee.enum.battery.prm_dyn.rc1  R1_mat=[.089, .076, .01; .042, .022, .099; .019, .007, .002; .051, .043, .029] Ohm  R1_vec=awgn(Rp, Parameter_noise) Ohm  tau1_mat=[44, 148, 235; 93, 110, 1000; 19, 27, 133; .5, 22, 3] s  tau1_vec=awgn(tau, Parameter_noise) s  R2_mat=[.014, .382, .407; .028, .006, .007; .014, .007, .006; .333, .956, .912] Ohm  R2_vec=[.382, .006, .007, .956] Ohm  tau2_mat=[1, 44, 5644; 11, 24, 506; 2, 14, 330; 3310, 13419, 30216] s  tau2_vec=[44, 24, 14, 13419] s  R3_mat=[.014, .382, .407; .028, .006, .007; .014, .007, .006; .333, .956, .912] Ohm  R3_vec=[.382, .006, .007, .956] Ohm  tau3_mat=[1, 44, 5644; 11, 24, 506; 2, 14, 330; 3310, 13419, 30216] s  tau3_vec=[44, 24, 14, 13419] s  R4_mat=[.014, .382, .407; .028, .006, .007; .014, .007, .006; .333, .956, .912] Ohm  R4_vec=[.382, .006, .007, .956] Ohm  tau4_mat=[1, 44, 5644; 11, 24, 506; 2, 14, 330; 3310, 13419, 30216] s  tau4_vec=[44, 24, 14, 13419] s  R5_mat=[.014, .382, .407; .028, .006, .007; .014, .007, .006; .333, .956, .912] Ohm  R5_vec=[.382, .006, .007, .956] Ohm  tau5_mat=[1, 44, 5644; 11, 24, 506; 2, 14, 330; 3310, 13419, 30216] s  tau5_vec=[44, 24, 14, 13419] s  prm_fade=ee.enum.battery.prm_fade.equations  N0=10  dV0=0  dR0=0  dAH=Capacity_deterioration  dRleak=0  dR1=0  dR2=0  dR3=0  dR4=0  dR5=0  N0vec=[100, 200, 300]  Tfadevec=[298.15, 323.15] K  dV0vec=[0, 0, 0]  dR0vec=[0, 0, 0]  dAHvec=[0, 0, 0]  dRleakvec=[0, 0, 0]  dR1vec=[0, 0, 0]  dR2vec=[0, 0, 0]  dR3vec=[0, 0, 0]  dR4vec=[0, 0, 0]  dR5vec=[0, 0, 0]  dV0mat=[0, 0; 0, 0; 0, 0]  dR0mat=[0, 0; 0, 0; 0, 0]  dAHmat=[0, 0; 0, 0; 0, 0]  dRleakmat=[0, 0; 0, 0; 0, 0]  dR1mat=[0, 0; 0, 0; 0, 0]  dR2mat=[0, 0; 0, 0; 0, 0]  dR3mat=[0, 0; 0, 0; 0, 0]  dR4mat=[0, 0; 0, 0; 0, 0]  dR5mat=[0, 0; 0, 0; 0, 0]  prm_age=ee.enum.battery.prm_age.disabled  prm_age_OCV=ee.enum.battery.prm_age_OCV.OCV  OCV_age=0.9  SOC_age=0.6  storage_dt_age_vec=[0] d  storage_T_age_vec=[273] K  OCV_scaling_age=2.2134e6  OCV_offset_age=1.632e6  temp_exp_age=0.515833569 V  t_exp_age=0.75  T_age_vec=[273.15, 298.15, 323.15] K  dt_age_vec=[90, 180, 270, 360] d  dR0_age_vec=[0, 0, 0]  t_meas_dR0_age=100 d  dR0_age_mat=[0, 0, 0; 0, 0, 0; 0, 0, 0; 0, 0, 0]  temperature=298.15 K  i_specify=off  i_priority=None  i=0 A  i_nominal_specify=off  i_nominal_unit=A  i_nominal_value=1  v_specify=off  v_priority=None  v=0 V  v_nominal_specify=off  v_nominal_unit=V  v_nominal_value=1  stateOfCharge_specify=on  stateOfCharge_priority=High  stateOfCharge=z0*1.3  stateOfCharge_nominal_specify=off  stateOfCharge_nominal_unit=1  stateOfCharge_nominal_value=1  num_cycles_specify=off  num_cycles_priority=High  num_cycles=0  num_cycles_nominal_specify=off  num_cycles_nominal_unit=1  num_cycles_nominal_value=1  thermal_mass=30000 J/K  temperature_specify=off  temperature_priority=High  temperature_nominal_specify=off  temperature_nominal_unit=K  temperature_nominal_value=1
      settings: SourceProductBaseCode=PS  InternalSimscapePortConfiguration="{\"Bottom\":[],\"Left\":[{\"id\":\"p\",\"label\":\"+\",\"type\":\"foundation.electrical.electrical\"},{\"id\":\"soc\",\"label\":\"SOC\",\"type\":\"output\"}],\"Right\":[{\"id\":\"n\",\"label\":\"-\",\"type\":\"foundation.electrical.electrical\"}],\"Top\":[]}"
  PS-Simulink Converter : nesl_utility/PS-Simulink Converter  PhysicalDomain=network_engine_domain  SubClassName=ps_output  LeftPortType=input  RightPortType=output  PseudoPeriodic=off  Frequencies=[]  Unit=inherit  AffineConversion=off
      settings: SourceProductBaseCode=PW,SS
  PS-Simulink Converter1 : nesl_utility/PS-Simulink Converter  PhysicalDomain=network_engine_domain  SubClassName=ps_output  LeftPortType=input  RightPortType=output  PseudoPeriodic=off  Frequencies=[]  Unit=inherit  AffineConversion=off
      settings: SourceProductBaseCode=PW,SS
  Selector : Selector  InputPortWidth=cell_count  IndexOptions=Index vector (dialog)  Indices=10  OutputSizes=1
  Simulink-PS Converter : nesl_utility/Simulink-PS Converter  PhysicalDomain=network_engine_domain  SubClassName=ps_input  LeftPortType=input  RightPortType=output  PseudoPeriodic=off  Frequencies=[]  NoiseDistribution=none  NoiseParameters=[]  Unit=1  AffineConversion=off  FilteringAndDerivatives=provide  SimscapeFilterOrder=1  InputFilterTimeConstant=0.001  UdotUserProvided=0
      settings: SourceProductBaseCode=PW,SS
  Switch : fl_lib/Electrical/Electrical Elements/Switch  R_closed=33 Ohm  G_open=1e-8 1/Ohm  Threshold=0.5  i_specify=off  i_priority=None  i=0 A  i_nominal_specify=off  i_nominal_unit=A  i_nominal_value=1  v_specify=off  v_priority=None  v=0 V  v_nominal_specify=off  v_nominal_unit=V  v_nominal_value=1
  Voltage Sensor : fl_lib/Electrical/Electrical Sensors/Voltage Sensor
  + : PMIOPort  Side=Left
  - : PMIOPort  Port=2  Side=Right
  SOC : Outport
  Voltage : Outport  Port=2
  wires:
  PS-Simulink Converter1/1 -> SOC/1
  PS-Simulink Converter/1 -> Voltage/1
  Balance/1 -> Selector/1
  Selector/1 -> Simulink-PS Converter/1
  connections:
  Battery (Table-Based)/LConn1 -- +/RConn1 -- Voltage Sensor/LConn1 -- Switch/LConn1
  PS-Simulink Converter/LConn1 -- Voltage Sensor/RConn1
  PS-Simulink Converter1/LConn1 -- Battery (Table-Based)/LConn2
  Battery (Table-Based)/RConn1 -- Switch/RConn2 -- -/RConn1 -- Voltage Sensor/RConn2
  Switch/RConn1 -- Simulink-PS Converter/RConn1
